simulink model "StopWatchStatechart_extended"  (Simulink 10.1)
settings: Solver=FixedStepAuto  StartTime=0.0  StopTime=1000.0  FixedStep=1e-3  RelTol=1e-3
settings Model: Creator=Lukas Bilal  LastModifiedBy=Lukas Bilal  EnablePacing=on
settings DataIOCC: SaveFormat=Dataset  ReturnWorkspaceOutputs=on
settings OptimizationCC: LifeSpan=auto
settings DebuggingCC: UnderspecifiedInitializationDetection=Simplified  MergeDetectMultiDrivingBlocksExec=error  SFUnexpectedBacktrackingDiag=error  SFNoUnconditionalDefaultTransitionDiag=error  SFExecutionAtInitializationDiag=warning  ArithmeticOperatorsInVariantConditions=error
settings HardwareCC: ProdBitPerPointer=64  ProdBitPerSizeT=64  ProdBitPerPtrDiffT=64  ProdLargestAtomicFloat=Float  ProdIntDivRoundTo=Zero  ProdEndianess=LittleEndian  ProdWordSize=64  ProdHWDeviceType=Intel->x86-64 (Windows64)
settings ModelReferenceCC: PropagateSignalLabelsOutOfModel=on
settings SFSimCC: SimUseLocalCustomCode=on  CustomCodeUndefinedFunction=FilterOut
settings RTWCC: RTWUseLocalCustomCode=on
settings CodeAppCC: StateflowObjectComments=off
settings GRTTargetCC: TargetLangStandard=C99 (ISO)  CombineOutputUpdateFcns=on  GRTInterface=off
settings ConfigComp: CovMetricSettings=dwe  CovHtmlReporting=off  CovSaveCumulativeToWorkspaceVar=off  CovSaveSingleToWorkspaceVar=off  CovExternalEMLEnable=on

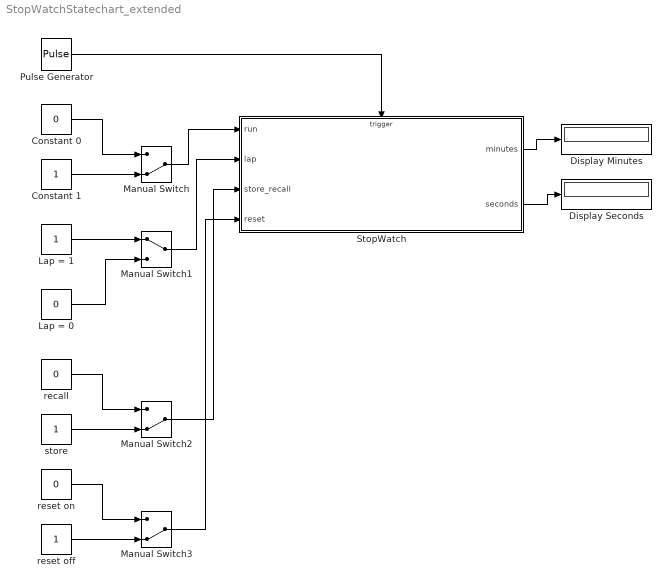
== system StopWatchStatechart_extended ==
  Constant 0 : Constant  Value=0  OutDataTypeStr=boolean
  Constant 1 : Constant  OutDataTypeStr=boolean
  Display Minutes : Display
  Display Seconds : Display
  Lap = 0 : Constant  Value=0  OutDataTypeStr=boolean
  Lap = 1 : Constant  OutDataTypeStr=boolean
  Manual Switch : ManualSwitch  CurrentSetting=0
  Manual Switch1 : ManualSwitch
  Manual Switch2 : ManualSwitch  CurrentSetting=0
  Manual Switch3 : ManualSwitch  CurrentSetting=0
  "Pulse Generator " : DiscretePulseGenerator  PulseType=Time based  Period=1  PulseWidth=5
  StopWatch : Stateflow chart  TreatAsAtomicUnit=on
  recall : Constant  Value=0  OutDataTypeStr=boolean
  reset off : Constant  OutDataTypeStr=boolean
  reset on : Constant  Value=0  OutDataTypeStr=boolean
  store : Constant  OutDataTypeStr=boolean
  wires:
  Constant 0/1 -> Manual Switch/1
  Constant 1/1 -> Manual Switch/2
  Manual Switch/1 -> StopWatch/1(run)
  StopWatch/1(minutes) -> Display Minutes/1
  StopWatch/2(seconds) -> Display Seconds/1
  Lap = 1/1 -> Manual Switch1/1
  Lap = 0/1 -> Manual Switch1/2
  Manual Switch1/1 -> StopWatch/2(lap)
  recall/1 -> Manual Switch2/1
  store/1 -> Manual Switch2/2
  "Pulse Generator "/1 -> StopWatch/Trigger
  Manual Switch2/1 -> StopWatch/3(store_recall)
  reset off/1 -> Manual Switch3/2
  reset on/1 -> Manual Switch3/1
  Manual Switch3/1 -> StopWatch/4(reset)

== stateflow chart StopWatch ==
  settings: executeAtInitialization=1
  state Stopped
    state Reset
    state Store
    state Recall
    (default) -> Recall
    Recall -> Reset [order 2] : [reset]
    Store -> Recall [order 1] : [store_recall] /
        | {
        |   minutes_intern = 0;
        |   seconds_intern = 0;
        |   seconds_stored = 0;
        |   minutes_stored = 0;
        | }
    Recall -> Store [order 1] : [store_recall] /
        | {
        |   minutes_stored = minutes_intern;
        |   seconds_stored = seconds_intern;
        | }
    Reset -> Reset : {
        |   seconds_stored = 0;
        |   minutes_stored = 0;
        | }
    Store -> Reset [order 2] : [reset]
  state Started
    state Lap [parallel]
      settings: executionOrder=3
      state lap
      (default) -> lap
      lap -> lap : [lap] /
          | {
          |   seconds = seconds_intern;
          |   minutes = minutes_intern;
          | }
    state Clock [parallel]
      settings: executionOrder=2
      state Counter
      (default) -> Counter
      Counter -> Counter [order 1] : after(1, clk) [seconds_intern < 59] /
          | {
          |   seconds_intern = seconds_intern + 1;
          | }
      Counter -> Counter [order 2] : after(1, clk) [seconds_intern == 59]
          | {
          |   minutes_intern = minutes_intern + 1;
          |   seconds_intern = 0;
          | }
    state store_recall [parallel]
      settings: executionOrder=1
      state store_recall
      (default) -> Started.store_recall.store_recall
      Started.store_recall.store_recall -> Started.store_recall.store_recall [order 1] : [store_recall && hasChanged(store_recall)]
          | {
          |   seconds_intern = seconds_stored;
          |   minutes_intern = minutes_stored;
          | }
      Started.store_recall.store_recall -> Started.store_recall.store_recall [order 2] : [~store_recall && hasChanged(store_recall)] /
          | {
          |   seconds_stored = seconds_intern;
          |   minutes_stored = minutes_intern;
          | }
  (default) -> Stopped
  Stopped -> Started : [run]
  Started -> Stopped : [~run]
  data: minutes output uint32 =uint32(0); seconds output uint8 =uint8(0); run input boolean; lap input boolean; minutes_intern local uint32 =uint32(0); seconds_intern local uint8 =uint8(0); seconds_stored local uint8 =uint8(0); minutes_stored local uint32 =uint32(0); store_recall input boolean; reset input boolean
  events: clk input RISING_EDGE_EVENT
